simulink model "cruise_control_top"  (Simulink 7.8)
settings: Solver=ode5  SolverMode=SingleTasking  StartTime=0.0  StopTime=50  FixedStep=0.01  RelTol=1e-3  AbsTol=1e-6
model workspace (MAT data in the model file):
  converter_data = [0  137.465208994  2.232; 0.1  137.065019157  2.075; 0.2  135.864449646  1.975; 0.3  135.664354728  1.846; 0.4  137.565256453  1.72; 0.5  140.366585312  1.564; 0.6  145.268910814  1.409; 0.7  152.872517717  1.254; 0.8  162.9773111  1.096; 0.81  164.27792807  1.08; 0.82  166.178829795  1.061; 0.83  167.979684062  1.043; 0.84  170.080680706  1.028; 0.85  172.781962105  1.012; 0.86  175.383196045  1.002; 0.87  179.585189333  1.002; 0.88  183.587087703  1.001; 0.89  189.890077635  0.998; 0.9  197.693779455  0.999; 0.92  215.902417037  1.001; 0.94  244.515990379  1.002]
  emap = [-40  -44  -49  -53  -57  -61  -65  -70  -74  -78  -82; 215  117  85  66  44  29  10  -2  -13  -22  -32; 245  208  178  148  122  104  85  66  48  33  18; 264  260  241  219  193  167  152  133  119  96  85; 264  279  282  275  260  238  223  208  189  171  152; 267  290  293  297  290  275  260  256  234  212  193; 267  297  305  305  305  301  293  282  267  249  226; 267  301  308  312  319  323  319  316  297  279  253; 267  301  312  319  327  327  327  327  312  293  267; 267  301  312  319  327  334  334  334  319  305  275]
  Iei = 0.0219914882836
  nevec = [800 1200 1600 2000 2400 2800 3200 3600 4000 4400 4800]
  p0 = 0.07934
  p1 = 0.07934
  thvec = [0; 20; 30; 40; 50; 60; 70; 80; 90; 100]
  vehicledata : num (value not decoded)
undefined symbols (not defined in the file or in its folder): sigbuilder_block
Description:
  | トップレベルモデル
settings Model: Creator=The MathWorks Inc.  LastModifiedBy=itoy  CovMetricSettings=dcmr  CovHTMLOptions=-aTS=1 -bRG=1 -bTC=1 -hTR=0 -nFC=0 -scm=1 -bcm=1 -xEv=0  CovModelRefEnable=off  ExtModeTrigMode=oneshot  ExtModeArmWhenConnect=off  ExtModeAutoUpdateStatusClock=off
settings DataIOCC: LimitDataPoints=off  SaveFormat=StructureWithTime  SaveOutput=off  SignalLogging=off  DSMLogging=off  SaveTime=off  SignalLoggingName=sigsOut
settings OptimizationCC: InlineParams=on  UseIntDivNetSlope=on  InlineInvariantSignals=on  InitFltsAndDblsToZero=on  EfficientMapNaN2IntZero=off  LifeSpan=1
settings DebuggingCC: SignalInfNanChecking=error  SaveWithParameterizedLinksMsg=none  CheckExecutionContextPreStartOutputMsg=on  CheckExecutionContextRuntimeOutputMsg=on  SolverPrmCheckMsg=none  MultiTaskDSMMsg=warning  MultiTaskCondExecSysMsg=none  IntegerOverflowMsg=error  FcnCallInpInsideContextMsg=Use local settings  BusObjectLabelMismatch=error  RootOutportRequireBusObject=error  StrictBusMsg=ErrorOnBusTreatedAsVector  BusNameAdapt=ErrorWithoutRepair  NonBusSignalsTreatedAsBus=error
settings HardwareCC: ProdIntDivRoundTo=Zero  ProdEndianess=LittleEndian  ProdHWDeviceType=NEC->V850  TargetUnknown=on
settings ModelReferenceCC: ModelReferenceNumInstancesAllowed=Single
settings SFSimCC: SFSimEcho=off  SimParseCustomCode=off
settings RTWCC: IncludeERTFirstTime=on
settings GRTTargetCC: TargetFcnLib=ansi_tfl_tmw.mat
settings ConfigComp: Description=Design Verifier Custom Configuration Component  DVMaxProcessTime=3000  DVModelCoverageObjectives=MCDC  DVMaxTestCaseSteps=500  DVTestSuiteOptimization=CombinedObjectives

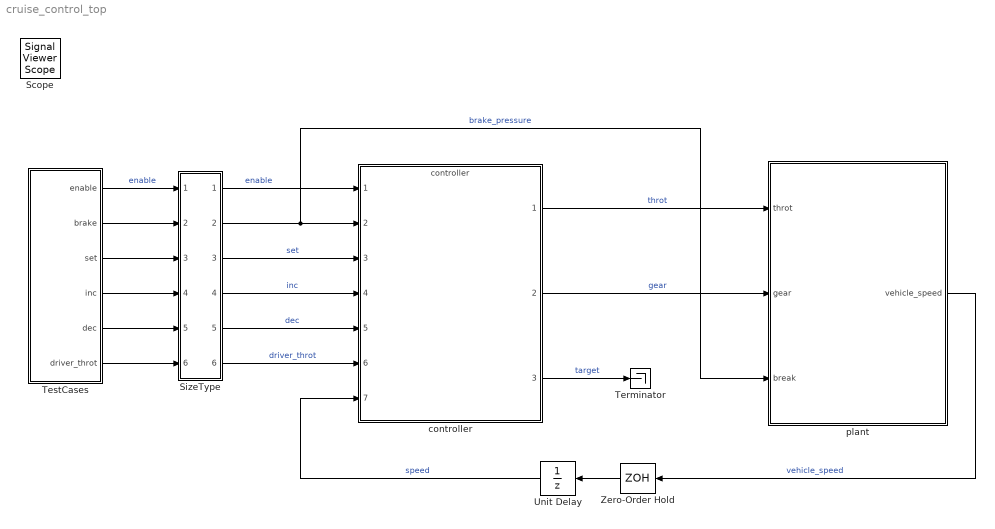
== system cruise_control_top ==
  SizeType : Subsystem
      mask Display: disp('')
  Terminator : Terminator
  TestCases : Subsystem  Tag=STV Subsys  LoadFcn=sigbuilder_block('load');  StartFcn=sigbuilder_block('start');  StopFcn=sigbuilder_block('stop');  ClipboardFcn=sigbuilder_block('clipboard');  mask(Sigbuilder block){}
      mask help: Create and generate interchangeable groups of signals whose waveforms are piecewise linear.
      mask init:
      | if ~strcmp(get_param(bdroot(gcbh),'SimulationStatus'),'stopped') tuvar = sigbuilder_block('maskInit'); end
      settings: CopyFcn=sigbuilder_block('copy');  DeleteFcn=sigbuilder_block('delete');  ModelCloseFcn=sigbuilder_block('modelClose');  PreSaveFcn=sigbuilder_block('preSave');  NameChangeFcn=sigbuilder_block('namechange');  OpenFcn=sigbuilder_block('open',[8.25 114 366.75 374.25 ]);  CloseFcn=sigbuilder_block('close');
      mask Display: plot(0,0,100,100,[10,10,40,40,10],[80,20,20,80,80],[40,10],[50,50], [40,27,10],[65,72,56],[40,25,25,10],[28,28,43,43]);
  Unit Delay : UnitDelay  SampleTime=-1
      settings: AttributesFormatString=<Init = %<X0>>
  Zero-Order Hold : ZeroOrderHold  SampleTime=0.01
  controller : ModelReference  ModelNameDialog=controller  SimulationMode=Normal  ModelReferenceVersion=1.215  CopyOfModelName=controller  DefaultDataLogging=off
  plant : Subsystem
  Scope : SignalViewerScope  IOType=viewer  NumInputPorts=4  RefreshTime=0.035000
      settings: TimeRange=50  YMin=0~0~0~1  YMax=60~5000~100~4
  wires:
  controller/2 -> plant/2(gear)  "gear"
  plant/1(vehicle_speed) -> Zero-Order Hold/1  "vehicle_speed"
  Unit Delay/1 -> controller/7  "speed"
  Zero-Order Hold/1 -> Unit Delay/1
  controller/1 -> plant/1(throt)  "throt"
  controller/3 -> Terminator/1  "target"
  SizeType/1(Out1) -> controller/1  "enable"
  SizeType/2(Out2) -> plant/3(break), controller/2  "brake_pressure"
  SizeType/3(Out3) -> controller/3  "set"
  SizeType/4(Out4) -> controller/4  "inc"
  SizeType/5(Out5) -> controller/5  "dec"
  SizeType/6(Out6) -> controller/6  "driver_throt"
  TestCases/1(enable) -> SizeType/1(In1)  "enable"
  TestCases/2(brake) -> SizeType/2(In2)
  TestCases/3(set) -> SizeType/3(In3)
  TestCases/4(inc) -> SizeType/4(In4)
  TestCases/5(dec) -> SizeType/5(In5)
  TestCases/6(driver_throt) -> SizeType/6(In6)

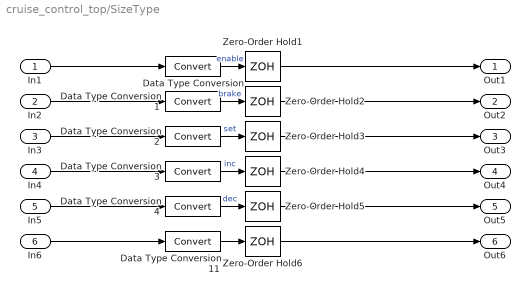
== system cruise_control_top/SizeType ==
  In1 : Inport
  In2 : Inport  Port=2
  In3 : Inport  Port=3
  In4 : Inport  Port=4
  In5 : Inport  Port=5
  In6 : Inport  Port=6
  Data Type Conversion{,1..4,11} (6 alike) : DataTypeConversion
  Zero-Order Hold{1..6} (6 alike) : ZeroOrderHold  SampleTime=0.01
  Out1 : Outport
  Out2 : Outport  Port=2
  Out3 : Outport  Port=3
  Out4 : Outport  Port=4
  Out5 : Outport  Port=5
  Out6 : Outport  Port=6
  wires:
  Data Type Conversion/1 -> Zero-Order Hold1/1  "enable"
  Data Type Conversion1/1 -> Zero-Order Hold2/1  "brake"
  Data Type Conversion2/1 -> Zero-Order Hold3/1  "set"
  Data Type Conversion3/1 -> Zero-Order Hold4/1  "inc"
  Data Type Conversion4/1 -> Zero-Order Hold5/1  "dec"
  In1/1 -> Data Type Conversion/1
  Zero-Order Hold1/1 -> Out1/1
  In2/1 -> Data Type Conversion1/1
  Zero-Order Hold2/1 -> Out2/1
  In3/1 -> Data Type Conversion2/1
  Zero-Order Hold3/1 -> Out3/1
  In4/1 -> Data Type Conversion3/1
  Zero-Order Hold4/1 -> Out4/1
  In5/1 -> Data Type Conversion4/1
  Zero-Order Hold5/1 -> Out5/1
  In6/1 -> Data Type Conversion11/1
  Zero-Order Hold6/1 -> Out6/1
  Data Type Conversion11/1 -> Zero-Order Hold6/1

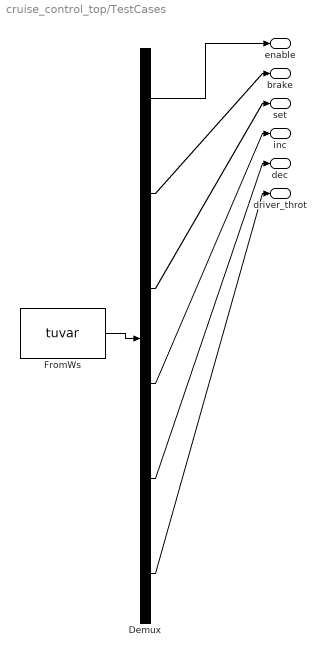
== system cruise_control_top/TestCases ==
  Demux : Demux  Tag=STV Demux  Outputs=6
  FromWs : FromWorkspace  Tag=STV FromWs  VariableName=tuvar  SampleTime=0  SigBuilderData=DataTag1  VnvData=DataTag2
      SigBuilderData=|
      | common.afterFinalStr = 'Extrapolate'
      | common.sampleTime = 0
      | dataSet(1).timeRange = [0 50]
      | dataSet(1).name = 'AccelBrake'
      | dataSet(2).timeRange = [0 50]
      | dataSet(2).name = 'ACC_Inc'
      | dataSet(3).timeRange = [0 50]
      | dataSet(3).name = 'ACC_Dec'
      | sbobj.Name = 'Signal Builder'
      | sbobj.Groups(1).Name = 'AccelBrake'
      | sbobj.Groups(1).Signals(1).Name = 'enable'
      | sbobj.Groups(1).Signals(1).XData = [0 10 25 40 50]
      | sbobj.Groups(1).Signals(1).YData = [0 0 0 0 0]
      | sbobj.Groups(1).Signals(2).Name = 'brake'
      | sbobj.Groups(1).Signals(2).XData = [0 10 25 25 40 50]
      | sbobj.Groups(1).Signals(2).YData = [0 0 0 1500 1500 1500]
      | sbobj.Groups(1).Signals(3).Name = 'set'
      | sbobj.Groups(1).Signals(3).XData = [0 10 25 25 40 50]
      | sbobj.Groups(1).Signals(3).YData = [0 0 0 0 0 0]
      | sbobj.Groups(1).Signals(4).Name = 'inc'
      | sbobj.Groups(1).Signals(4).XData = [0 10 25 25 40 50]
      | sbobj.Groups(1).Signals(4).YData = [0 0 0 0 0 0]
      | sbobj.Groups(1).Signals(5).Name = 'dec'
      | sbobj.Groups(1).Signals(5).XData = [0 10 25 25 40 50]
      | sbobj.Groups(1).Signals(5).YData = [0 0 0 0 0 0]
      | sbobj.Groups(1).Signals(6).Name = 'driver_throt'
      | sbobj.Groups(1).Signals(6).XData = [0 10 25 25 40 50]
      | sbobj.Groups(1).Signals(6).YData = [100 100 0 0 0 0]
      | sbobj.Groups(1).TimeRange = [0 50]
      | sbobj.Groups(2).Name = 'ACC_Inc'
      | sbobj.Groups(2).Signals(1).Name = 'enable'
      | sbobj.Groups(2).Signals(1).XData = [0 10 20 30 40 50]
      | sbobj.Groups(2).Signals(1).YData = [1 1 1 1 1 1]
      | sbobj.Groups(2).Signals(2).Name = 'brake'
      | sbobj.Groups(2).Signals(2).XData = [0 10 20 20 30 30 40 40 50]
      | sbobj.Groups(2).Signals(2).YData = [0 0 0 0 0 0 0 0 0]
      | sbobj.Groups(2).Signals(3).Name = 'set'
      | sbobj.Groups(2).Signals(3).XData = [0 10 20 20 30 30 40 40 50]
      | sbobj.Groups(2).Signals(3).YData = [0 0 0 1 1 0 0 0 0]
      | sbobj.Groups(2).Signals(4).Name = 'inc'
      | sbobj.Groups(2).Signals(4).XData = [0 10 20 20 30 30 40 40 50]
      | sbobj.Groups(2).Signals(4).YData = [0 0 0 0 0 1 1 0 0]
      | sbobj.Groups(2).Signals(5).Name = 'dec'
      | sbobj.Groups(2).Signals(5).XData = [0 10 20 20 30 30 40 40 50]
      | sbobj.Groups(2).Signals(5).YData = [0 0 0 0 0 0 0 0 0]
      | sbobj.Groups(2).Signals(6).Name = 'driver_throt'
      | sbobj.Groups(2).Signals(6).XData = [0 10 20 20 30 30 40 40 50]
      | sbobj.Groups(2).Signals(6).YData = [100 100 100 0 0 0 0 0 0]
      | sbobj.Groups(2).TimeRange = [0 50]
      | sbobj.Groups(3).Name = 'ACC_Dec'
      | sbobj.Groups(3).Signals(1).Name = 'enable'
      | sbobj.Groups(3).Signals(1).XData = [0 10 20 30 40 50]
      | sbobj.Groups(3).Signals(1).YData = [1 1 1 1 1 1]
      | sbobj.Groups(3).Signals(2).Name = 'brake'
      | sbobj.Groups(3).Signals(2).XData = [0 10 20 20 30 30 40 40 50]
      | sbobj.Groups(3).Signals(2).YData = [0 0 0 0 0 0 0 0 0]
      | sbobj.Groups(3).Signals(3).Name = 'set'
      | sbobj.Groups(3).Signals(3).XData = [0 10 20 20 30 30 40 40 50]
      | sbobj.Groups(3).Signals(3).YData = [0 0 0 1 1 0 0 0 0]
      | sbobj.Groups(3).Signals(4).Name = 'inc'
      | sbobj.Groups(3).Signals(4).XData = [0 10 20 20 30 30 40 40 50]
      | sbobj.Groups(3).Signals(4).YData = [0 0 0 0 0 0 0 0 0]
      | sbobj.Groups(3).Signals(5).Name = 'dec'
      | sbobj.Groups(3).Signals(5).XData = [0 10 20 20 30 30 40 40 50]
      | sbobj.Groups(3).Signals(5).YData = [0 0 0 0 0 1 1 0 0]
      | sbobj.Groups(3).Signals(6).Name = 'driver_throt'
      | sbobj.Groups(3).Signals(6).XData = [0 10 20 20 30 30 40 40 50]
      | sbobj.Groups(3).Signals(6).YData = [100 100 100 0 0 0 0 0 0]
      | sbobj.Groups(3).TimeRange = [0 50]
  enable : Outport  Tag=STV Outport
  brake : Outport  Tag=STV Outport  Port=2
  set : Outport  Tag=STV Outport  Port=3
  inc : Outport  Tag=STV Outport  Port=4
  dec : Outport  Tag=STV Outport  Port=5
  driver_throt : Outport  Tag=STV Outport  Port=6
  wires:
  Demux/1 -> enable/1
  FromWs/1 -> Demux/1
  Demux/2 -> brake/1
  Demux/3 -> set/1
  Demux/4 -> inc/1
  Demux/5 -> dec/1
  Demux/6 -> driver_throt/1

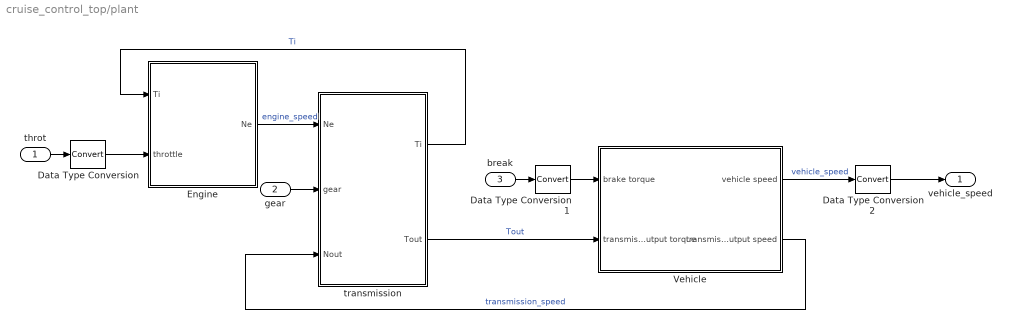
== system cruise_control_top/plant ==
  throt : Inport
  gear : Inport  Port=2
  break : Inport  Port=3
  Data Type Conversion : DataTypeConversion
  Data Type Conversion1 : DataTypeConversion
  Data Type Conversion2 : DataTypeConversion
  Engine : Subsystem
  Vehicle : Subsystem  mask(vehicle model){Rfd=vehicledata(1), rload0=vehicledata(2), rload2=vehicledata(3), Rw=vehicledata(4), Iv=vehicledata(5), N20=vehicledata(6)/vehicledata(4)*vehicledata(1)}
      mask prompts: Rfd "final drive ratio"; rload0 "drag friction at wheels"; rload2 "aerodynamic drag"; Rw "wheel radius"; Iv "vehicle inertia"; N20 "initial transmission output speed"
      mask help: vehicle dynamics: torque input from trans., outputs are input speed (transmission output) and vehicle speed
      mask Display: image(imread([matlabroot,'/toolbox/simulink/simdemos/automotive/html/NSX_3Colors.jpg']))
  transmission : Subsystem
  vehicle_speed : Outport
  wires:
  transmission/1(Ti) -> Engine/1(Ti)  "Ti"
  Engine/1(Ne) -> transmission/1(Ne)  "engine_speed"
  transmission/2(Tout) -> Vehicle/2(transmission output torque)  "Tout"
  Vehicle/2(transmission output speed) -> transmission/3(Nout)  "transmission_speed"
  throt/1 -> Data Type Conversion/1
  break/1 -> Data Type Conversion1/1
  Vehicle/1(vehicle speed) -> Data Type Conversion2/1  "vehicle_speed"
  gear/1 -> transmission/2(gear)
  Data Type Conversion/1 -> Engine/2(throttle)
  Data Type Conversion1/1 -> Vehicle/1(brake torque)
  Data Type Conversion2/1 -> vehicle_speed/1

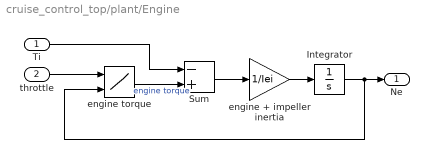
== system cruise_control_top/plant/Engine ==
  Ti : Inport
  throttle : Inport  Port=2
  Integrator : Integrator  InitialCondition=1000  LimitOutput=on  UpperSaturationLimit=6000  LowerSaturationLimit=600  ZeroCross=off
  Sum : Sum  Inputs=-+  SaturateOnIntegerOverflow=on  InputSameDT=on  OutDataTypeStr=Inherit: Same as first input
  engine torque : Lookup2D  RowIndex=thvec*0.3  ColumnIndex=nevec  Table=emap  InputSameDT=on
  engine + impeller inertia : Gain  Gain=1/Iei  SaturateOnIntegerOverflow=on  OutDataTypeStr=Inherit: Same as input  ParamDataTypeStr=Inherit: Same as input
  Ne : Outport  InitialOutput=0
  wires:
  Ti/1 -> Sum/1
  throttle/1 -> engine torque/1
  Integrator/1 -> engine torque/2, Ne/1
  Sum/1 -> engine + impeller inertia/1
  engine + impeller inertia/1 -> Integrator/1
  engine torque/1 -> Sum/2  "engine torque"

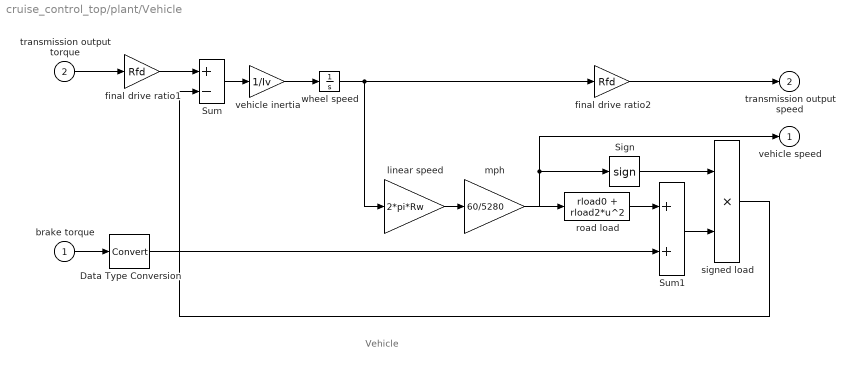
== system cruise_control_top/plant/Vehicle ==
  note: Vehicle
  brake torque : Inport
  transmission output torque : Inport  Port=2
  Data Type Conversion : DataTypeConversion
  Sign : Signum
  Sum : Sum  Inputs=+-  SaturateOnIntegerOverflow=on  InputSameDT=on  OutDataTypeStr=Inherit: Same as first input
  Sum1 : Sum  SaturateOnIntegerOverflow=on  InputSameDT=on  OutDataTypeStr=Inherit: Same as first input
  final drive ratio1 : Gain  Gain=Rfd  SaturateOnIntegerOverflow=on  OutDataTypeStr=Inherit: Same as input  ParamDataTypeStr=Inherit: Same as input
  final drive ratio2 : Gain  Gain=Rfd  SaturateOnIntegerOverflow=on  OutDataTypeStr=Inherit: Same as input  ParamDataTypeStr=Inherit: Same as input
  linear speed : Gain  Gain=2*pi*Rw  SaturateOnIntegerOverflow=on  OutDataTypeStr=Inherit: Same as input  ParamDataTypeStr=Inherit: Same as input
  mph : Gain  Gain=60/5280  SaturateOnIntegerOverflow=on  OutDataTypeStr=Inherit: Same as input  ParamDataTypeStr=Inherit: Same as input
  road load : Fcn  Expr=rload0 + rload2*u^2
  signed load : Product  SaturateOnIntegerOverflow=on  InputSameDT=on  OutDataTypeStr=Inherit: Same as first input
  vehicle inertia : Gain  Gain=1/Iv  SaturateOnIntegerOverflow=on  OutDataTypeStr=Inherit: Same as input  ParamDataTypeStr=Inherit: Same as input
  wheel speed : Integrator  InitialCondition=N20/Rfd  ZeroCross=off
  vehicle speed : Outport  InitialOutput=0
  transmission output speed : Outport  Port=2  InitialOutput=0
  wires:
  final drive ratio2/1 -> transmission output speed/1
  brake torque/1 -> Data Type Conversion/1
  Sum1/1 -> signed load/2
  road load/1 -> Sum1/1
  Sign/1 -> signed load/1
  signed load/1 -> Sum/2
  transmission output torque/1 -> final drive ratio1/1
  vehicle inertia/1 -> wheel speed/1
  Sum/1 -> vehicle inertia/1
  mph/1 -> vehicle speed/1, Sign/1, road load/1
  linear speed/1 -> mph/1
  wheel speed/1 -> linear speed/1, final drive ratio2/1
  final drive ratio1/1 -> Sum/1
  Data Type Conversion/1 -> Sum1/2

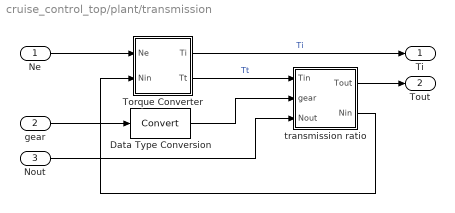
== system cruise_control_top/plant/transmission ==
  Ne : Inport
  gear : Inport  Port=2
  Nout : Inport  Port=3
  Data Type Conversion : DataTypeConversion
  Torque Converter : Subsystem  mask(torque converter){speedratio=converter_data(:,1), Kfactor=converter_data(:,2), Torkratio=converter_data(:,3)}
      mask prompts: speedratio "speed ratio"; Kfactor "K factor"; Torkratio "torque ratio"
      mask help: torque converter
      mask Help: Torque converter input and output torques are computed as a function of the input and output speeds
      mask Display: plot([cos([90:10:450]*pi/180),.63*cos([90:10:450]*pi/180),.63*cos([90:10:240]*pi/180),cos([240:10:300]*pi/180),.63*cos([300]*pi/180)],[sin([90:10:450]*pi/180),.63*sin([90:10:450]*pi/180)+.1,.63*sin([90:10:240]*pi/180)+.1,sin([240:10:300]*pi/180),.63*sin([300]*pi/180)+.1])
  transmission ratio : Subsystem
  Ti : Outport  InitialOutput=0
  Tout : Outport  Port=2  InitialOutput=0
  wires:
  transmission ratio/1(Tout) -> Tout/1
  Torque Converter/1(Ti) -> Ti/1  "Ti"
  Nout/1 -> transmission ratio/3(Nout)
  gear/1 -> Data Type Conversion/1
  Ne/1 -> Torque Converter/1(Ne)
  transmission ratio/2(Nin) -> Torque Converter/2(Nin)
  Torque Converter/2(Tt) -> transmission ratio/1(Tin)  "Tt"
  Data Type Conversion/1 -> transmission ratio/2(gear)

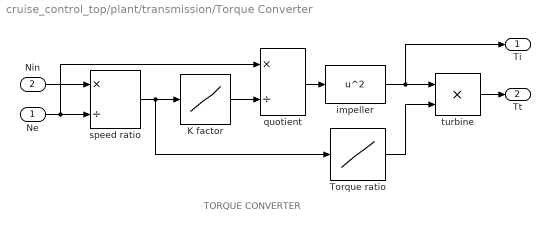
== system cruise_control_top/plant/transmission/Torque Converter ==
  note: TORQUE CONVERTER
  Ne : Inport
  Nin : Inport  Port=2
  K factor : Lookup  InputValues=speedratio  Table=Kfactor  SaturateOnIntegerOverflow=on
  Torque ratio : Lookup  InputValues=speedratio  Table=Torkratio  SaturateOnIntegerOverflow=on
  impeller : Fcn  Expr=u^2
  quotient : Product  Inputs=*/  SaturateOnIntegerOverflow=on  InputSameDT=on  OutDataTypeStr=Inherit: Same as first input
  speed ratio : Product  Inputs=*/  SaturateOnIntegerOverflow=on  InputSameDT=on  OutDataTypeStr=Inherit: Same as first input
  turbine : Product  SaturateOnIntegerOverflow=on  InputSameDT=on  OutDataTypeStr=Inherit: Same as first input
  Ti : Outport  InitialOutput=0
  Tt : Outport  Port=2  InitialOutput=0
  wires:
  Torque ratio/1 -> turbine/2
  quotient/1 -> impeller/1
  K factor/1 -> quotient/2
  speed ratio/1 -> Torque ratio/1, K factor/1
  impeller/1 -> turbine/1, Ti/1
  turbine/1 -> Tt/1
  Ne/1 -> speed ratio/2, quotient/1
  Nin/1 -> speed ratio/1

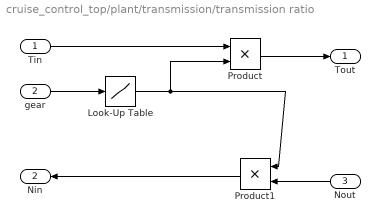
== system cruise_control_top/plant/transmission/transmission ratio ==
  Tin : Inport
  gear : Inport  Port=2
  Nout : Inport  Port=3
  Look-Up Table : Lookup  InputValues=[1 2 3 4]  Table=[2.393 1.450 1.000 0.677]  SaturateOnIntegerOverflow=on
  Product : Product  SaturateOnIntegerOverflow=on  InputSameDT=on  OutDataTypeStr=Inherit: Same as first input
  Product1 : Product  SaturateOnIntegerOverflow=on  InputSameDT=on  OutDataTypeStr=Inherit: Same as first input
  Tout : Outport  InitialOutput=0
  Nin : Outport  Port=2  InitialOutput=0
  wires:
  Look-Up Table/1 -> Product1/1, Product/2
  Nout/1 -> Product1/2
  Product1/1 -> Nin/1
  Product/1 -> Tout/1
  Tin/1 -> Product/1
  gear/1 -> Look-Up Table/1
